simulink library "annVolume"  (R2022b)
settings: Solver=VariableStepAuto  StartTime=0.0  StopTime=10.0  RelTol=1e-3
undefined symbols (not defined in the file or in its folder): num_inp_chs
libraries: AnnVolumeBtc x1
settings Model: Creator=kl13806  LastModifiedBy=kl13806
settings SolverCC: AlgebraicLoopSolver=TrustRegion
settings DebuggingCC: UnconnectedInputMsg=warning  UnconnectedOutputMsg=warning  UnconnectedLineMsg=warning  SFMachineParentedDataDiag=warning  ArithmeticOperatorsInVariantConditions=warning
settings ModelReferenceCC: EnableRefExpFcnMdlSchedulingChecks=on
settings SFSimCC: SimUseLocalCustomCode=off  CustomCodeUndefinedFunction=UseInterfaceOnly
settings RTWCC: RTWUseLocalCustomCode=off  DLArmComputeVersion=19.05

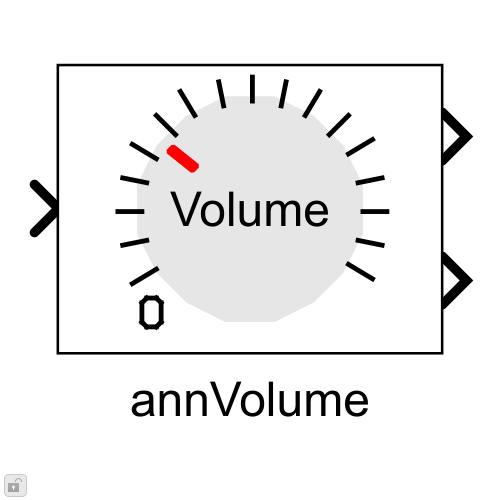
[thumbnail: Simulink's stored preview of the top-level diagram]
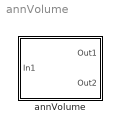
== system annVolume ==
  annVolume : Subsystem  mask(Bose Audio Volume){MaskVolumeName=Volume, initial_linear_gain=ones(1,num_inp_chs), num_inp_chs=num_inp_chs, LastName=0, PackageName=, BankNumber=[], TriggerInit=[325 175 405 235]}
      mask prompts: MaskVolumeName "Signal Name (controls FeaturePath)"; initial_linear_gain "Initial gain (linear)"; num_inp_chs "Number of i/p channels"; PackageName "Tuning Package"; BankNumber "Memory Bank Number:"; TriggerInit "Hidden: MoveFcn redraw"
      mask help: This volume signal block includes receipt of volume level (via RTC) as well as tuning variables to calibrate a gain table that maps 8-bit integer volume index (from RTC) to float decibels.
      mask init:
      | blkh = gcbh;
      | % Copy discrete mask parameters into a classdef object
      | InnerLinkConfig = AnnVolumeConfig;
      | InnerLinkConfig.InitialLinearGain = initial_linear_gain;
      | InnerLinkConfig.NumInputChannels = num_inp_chs;
      | InnerLinkConfig.BankNumber = BankNumber;
      settings: MoveFcn=VolumeMask.CB_TriggerInit(gcbh);
      mask TypeOptions MaskVolumeName: InnerLink/FeatureName
      mask TypeOptions PackageName: InnerLink/PackageName
      mask Callback TriggerInit: VolumeMask.CB_TriggerInit(gcbh);
      mask DialogControl CalibrationGroup Prompt: Signal Calibration
      mask Display:
      | [path,w,h] = IconVolumeMask();
      | 
      | % work in pixels since the icon does not scale
      | pos = get(gcbh,'position');
      | bw = pos(3) - pos(1);
      | bh = pos(4) - pos(2);
      | 
      | % Draw centered icon
      | xAdj = bw/2 - w/2;
      | yAdj = bh/2 - h/2;
      | for i=1:length(path)
      |     if (path(i).rgb(1) >= 0)
      |         patch(path(i).x+xAdj, path(i).y+yAdj, path(i).rgb);
      |     end
      |     if (path(i).stroke(1) >= 0)
      |         plot(path(i).x+xAdj, path(i).y+yAdj);
      |     end
      | end
      | 
      | % Display some text
      | text(bw/2, bh/2,MaskVolumeName, ...
      |     'horizontalAlignment','center', ...
      |     'VerticalAlignment','middle');

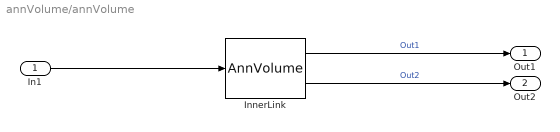
== system annVolume/annVolume ==
  In1 : Inport
  InnerLink : AnnVolumeBtc/AnnVolume  FeatureName=Volume  Config=InnerLinkConfig  TriggerInit=[815 415 895 475]
      settings: SourceProductName=Bose Blocklib
  Out1 : Outport
  Out2 : Outport  Port=2
  wires:
  InnerLink/1 -> Out1/1  "Out1"
  InnerLink/2 -> Out2/1  "Out2"
  In1/1 -> InnerLink/1
